simulink model "Lab22021a"  (R2021a)
settings: Solver=VariableStepAuto  StartTime=0.0  StopTime=70  RelTol=1e-3
libraries: simulink x4
settings Model: Creator=sarah  LastModifiedBy=sarah
settings DebuggingCC: UnconnectedInputMsg=none  UnconnectedOutputMsg=none  UnconnectedLineMsg=none
settings RTWCC: DLArmComputeVersion=20.02.1

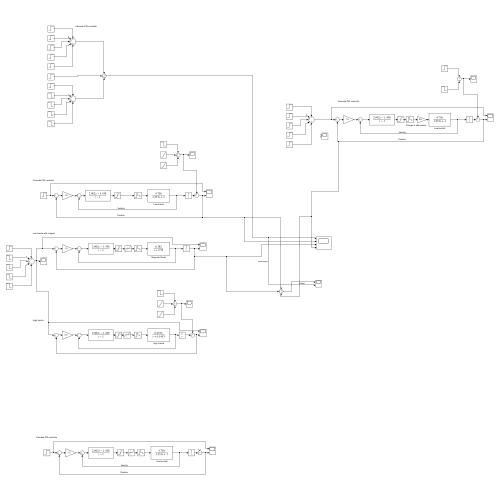
[thumbnail: Simulink's stored preview of the top-level diagram]
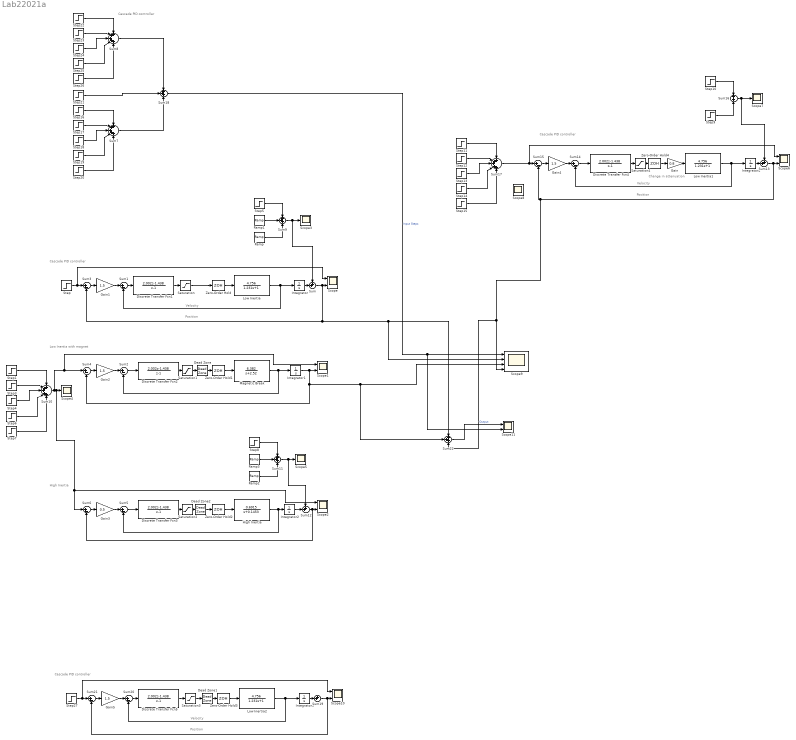
== system Lab22021a ==
  note: Change in attenuation
  note: Position
  note: Velocity
  note: Cascade PID controller
  note: Low Inertia with magnet
  note: High Inertia
  note: Position
  note: Cascade PID controller
  note: Velocity
  note: Cascade PID controller
  note: Position
  note: Velocity
  note: Cascade PID controller
  Dead Zone : DeadZone  LowerValue=-1.53  UpperValue=0.39  SaturateOnIntegerOverflow=on
  Dead Zone1 : DeadZone  LowerValue=-1.48  UpperValue=00.39  SaturateOnIntegerOverflow=on
  Dead Zone2 : DeadZone  LowerValue=-0.49  UpperValue=0.43  SaturateOnIntegerOverflow=on
  Discrete Transfer Fcn{1..5} (5 alike) : DiscreteTransferFcn  Numerator=[2.002 -1.438]  Denominator=[1 -1]  SampleTime=0.05
  Gain : Gain  Gain=0.8
  Gain{1..2,4..5} (4 alike) : Gain  Gain=1.5
  Gain3 : Gain  Gain=0.5
  High Inertia : TransferFcn  Numerator=[0.6915]  Denominator=[1 0.1453]
  Integrator{,1..4} (5 alike) : Integrator
  Low Inertia : TransferFcn  Numerator=[4.756]  Denominator=[1.231 1]
  Low Inertia1 : TransferFcn  Numerator=[4.756]  Denominator=[1.231 1]
  Low Inertia2 : TransferFcn  Numerator=[4.756]  Denominator=[1.231 1]
  Magnetic Break : TransferFcn  Numerator=[6.382]  Denominator=[1 2.52]
  Ramp : simulink/Sources/Ramp  slope=0.8  start=12.5  InitialOutput=0
  Ramp1 : simulink/Sources/Ramp  slope=-0.8  start=15  InitialOutput=0
  Ramp2 : simulink/Sources/Ramp  slope=0.8  start=12.5  InitialOutput=0
  Ramp3 : simulink/Sources/Ramp  slope=-0.8  start=15  InitialOutput=0
  Saturation{,1..4} (5 alike) : Saturate  UpperLimit=+10  LowerLimit=-10
  Scope{,1..2,6,10..11} (6 alike) : Scope  NumInputPorts=2
  Scope{3..5,7..8} (5 alike) : Scope
  Scope9 : Scope  NumInputPorts=4
  Step : Step  Time=5  After=5  SampleTime=0
  Step1 : Step  Time=32.9  After=2  SampleTime=0
  Step10 : Step  Time=49  After=0.8  SampleTime=0
  Step11 : Step  Time=46  SampleTime=0
  Step12 : Step  Time=51.5  After=2.2  SampleTime=0
  Step13 : Step  Time=53  After=2.8  SampleTime=0
  Step14 : Step  Time=54  After=3  SampleTime=0
  Step15 : Step  Time=59  After=1.6  SampleTime=0
  Step16 : Step  Time=32.9  After=2  SampleTime=0
  Step17 : Step  Time=35  After=-3.2  SampleTime=0
  Step18 : Step  Time=36.5  After=-2.6  SampleTime=0
  Step19 : Step  Time=39  After=-2.8  SampleTime=0
  Step20 : Step  Time=40  After=-4  SampleTime=0
  Step21 : Step  Time=5  After=5  SampleTime=0
  Step22 : Step  Time=46  SampleTime=0
  Step23 : Step  Time=51.5  After=2.2  SampleTime=0
  Step24 : Step  Time=53  After=2.8  SampleTime=0
  Step25 : Step  Time=54  After=3  SampleTime=0
  Step26 : Step  Time=59  After=1.6  SampleTime=0
  Step27 : Step  Time=5  After=5  SampleTime=0
  Step3 : Step  Time=35  After=-3.2  SampleTime=0
  Step4 : Step  Time=36.5  After=-2.6  SampleTime=0
  Step5 : Step  Time=15  After=-2  SampleTime=0
  Step6 : Step  Time=39  After=-2.8  SampleTime=0
  Step7 : Step  Time=40  After=-4  SampleTime=0
  Step8 : Step  Time=15  After=-2  SampleTime=0
  Step9 : Step  Time=49.1  After=-0.8  SampleTime=0
  Sum{,12..13,19} (4 alike) : Sum  Inputs=++|
  Sum{1..6,14..15,20..21} (10 alike) : Sum  Inputs=|+-
  Sum{7..8,10,17} (4 alike) : Sum  Inputs=+++++
  Sum{9,11,18,22} (4 alike) : Sum  Inputs=+++
  Sum16 : Sum
  Zero-Order Hold{,1,3..4} (4 alike) : ZeroOrderHold  SampleTime=0.05
  Zero-Order Hold2 : ZeroOrderHold  SampleTime=0.02
  wires:
  Sum1/1 -> Discrete Transfer Fcn1/1
  Discrete Transfer Fcn1/1 -> Saturation/1
  Sum3/1 -> Gain1/1
  Step/1 -> Sum3/1, Scope/1
  Zero-Order Hold/1 -> Low Inertia/1
  Gain1/1 -> Sum1/1
  Gain2/1 -> Sum2/1
  Zero-Order Hold1/1 -> Magnetic Break/1
  Discrete Transfer Fcn2/1 -> Saturation1/1
  Integrator1/1 -> Sum22/2, Scope9/3, Sum4/2, Scope1/2
  Sum4/1 -> Gain2/1
  Sum2/1 -> Discrete Transfer Fcn2/1
  Magnetic Break/1 -> Sum2/2, Integrator1/1
  Gain3/1 -> Sum5/1
  Zero-Order Hold2/1 -> High Inertia/1
  Discrete Transfer Fcn3/1 -> Saturation2/1
  Sum6/1 -> Gain3/1
  Step7/1 -> Sum10/5
  Sum5/1 -> Discrete Transfer Fcn3/1
  High Inertia/1 -> Sum5/2, Integrator2/1
  Low Inertia/1 -> Integrator/1, Sum1/2
  Sum9/1 -> Sum/1, Scope3/1
  Ramp/1 -> Sum9/3
  Ramp1/1 -> Sum9/2
  Integrator/1 -> Sum/2
  Sum/1 -> Sum22/1, Scope9/2, Sum3/2, Scope/2
  Step5/1 -> Sum9/1
  Step1/1 -> Sum10/1
  Step3/1 -> Sum10/2
  Step4/1 -> Sum10/3
  Step6/1 -> Sum10/4
  Sum10/1 -> Scope1/1, Sum4/1, Scope2/1, Sum6/1, Scope4/1
  Ramp2/1 -> Sum11/3
  Ramp3/1 -> Sum11/2
  Step8/1 -> Sum11/1
  Sum11/1 -> Sum12/1, Scope5/1
  Integrator2/1 -> Sum12/2
  Sum12/1 -> Sum6/2, Scope2/2
  Step10/1 -> Sum16/1
  Step15/1 -> Sum17/5
  Zero-Order Hold4/1 -> Gain/1
  Gain/1 -> Low Inertia1/1
  Sum15/1 -> Gain4/1
  Step9/1 -> Sum16/2
  Discrete Transfer Fcn4/1 -> Saturation4/1
  Sum14/1 -> Discrete Transfer Fcn4/1
  Low Inertia1/1 -> Integrator4/1, Sum14/2
  Gain4/1 -> Sum14/1
  Sum17/1 -> Sum15/1, Scope6/1
  Saturation4/1 -> Zero-Order Hold4/1
  Sum13/1 -> Sum22/3, Scope9/4, Sum15/2, Scope6/2
  Step13/1 -> Sum17/3
  Step14/1 -> Sum17/4
  Integrator4/1 -> Sum13/2
  Step12/1 -> Sum17/2
  Sum16/1 -> Sum13/1, Scope7/1
  Step11/1 -> Sum17/1
  Step17/1 -> Sum7/2
  Step20/1 -> Sum7/5
  Step16/1 -> Sum7/1
  Step19/1 -> Sum7/4
  Step18/1 -> Sum7/3
  Step22/1 -> Sum8/1
  Step24/1 -> Sum8/3
  Step23/1 -> Sum8/2
  Step26/1 -> Sum8/5
  Step25/1 -> Sum8/4
  Step21/1 -> Sum18/2
  Sum8/1 -> Sum18/1
  Sum7/1 -> Sum18/3
  Sum18/1 -> Scope11/2, Scope9/1  "Input Steps"
  Sum21/1 -> Gain5/1
  Dead Zone1/1 -> Zero-Order Hold3/1
  Zero-Order Hold3/1 -> Low Inertia2/1
  Sum20/1 -> Discrete Transfer Fcn5/1
  Low Inertia2/1 -> Integrator3/1, Sum20/2
  Discrete Transfer Fcn5/1 -> Saturation3/1
  Step27/1 -> Sum21/1, Scope10/1
  Integrator3/1 -> Sum19/2
  Saturation3/1 -> Dead Zone1/1
  Sum19/1 -> Sum21/2, Scope10/2
  Gain5/1 -> Sum20/1
  Saturation1/1 -> Dead Zone/1
  Dead Zone/1 -> Zero-Order Hold1/1
  Saturation2/1 -> Dead Zone2/1
  Dead Zone2/1 -> Zero-Order Hold2/1
  Saturation/1 -> Zero-Order Hold/1
  Sum22/1 -> Scope11/1  "Output"
